simulink model "thrust_torque"  (R2025b)
settings: Solver=VariableStepAuto  StartTime=0.0  StopTime=10.0  RelTol=1e-3
settings Model: Creator=BillL  LastModifiedBy=BillL

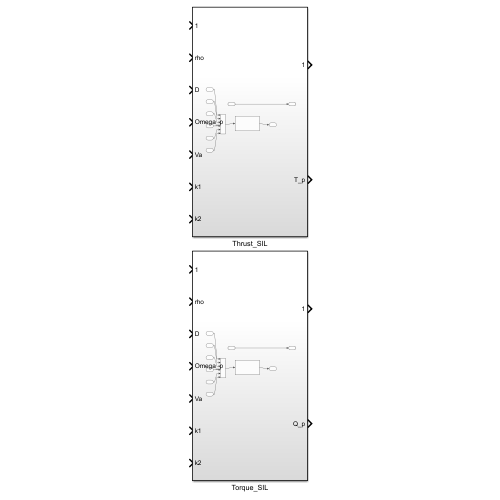
[thumbnail: Simulink's stored preview of the top-level diagram]
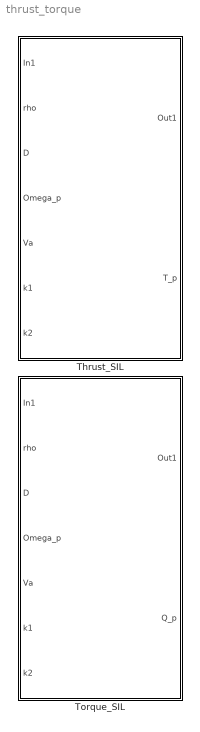
== system thrust_torque ==
  Thrust_SIL : Subsystem
  Torque_SIL : Subsystem

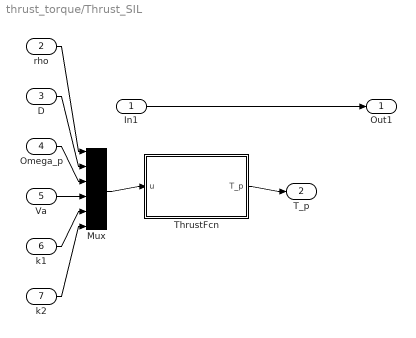
== system thrust_torque/Thrust_SIL ==
  In1 : Inport
  rho : Inport  Port=2
  D : Inport  Port=3
  Omega_p : Inport  Port=4
  Va : Inport  Port=5
  k1 : Inport  Port=6
  k2 : Inport  Port=7
  Mux : Mux  Inputs=6
  ThrustFcn : MATLAB Function  TreatAsAtomicUnit=on
  Out1 : Outport
  T_p : Outport  Port=2
  wires:
  In1/1 -> Out1/1
  rho/1 -> Mux/1
  D/1 -> Mux/2
  Omega_p/1 -> Mux/3
  Va/1 -> Mux/4
  k1/1 -> Mux/5
  k2/1 -> Mux/6
  Mux/1 -> ThrustFcn/1(u)
  ThrustFcn/1(T_p) -> T_p/1

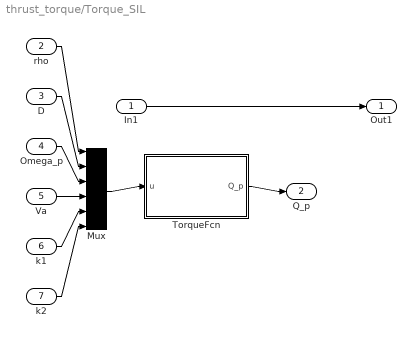
== system thrust_torque/Torque_SIL ==
  In1 : Inport
  rho : Inport  Port=2
  D : Inport  Port=3
  Omega_p : Inport  Port=4
  Va : Inport  Port=5
  k1 : Inport  Port=6
  k2 : Inport  Port=7
  Mux : Mux  Inputs=6
  TorqueFcn : MATLAB Function  TreatAsAtomicUnit=on
  Out1 : Outport
  Q_p : Outport  Port=2
  wires:
  In1/1 -> Out1/1
  rho/1 -> Mux/1
  D/1 -> Mux/2
  Omega_p/1 -> Mux/3
  Va/1 -> Mux/4
  k1/1 -> Mux/5
  k2/1 -> Mux/6
  Mux/1 -> TorqueFcn/1(u)
  TorqueFcn/1(Q_p) -> Q_p/1

== matlab function thrust_torque/Thrust_SIL/ThrustFcn ==
  data: u input; T_p output
function T_p = thrust_block(u)
rho = u(1); D = u(2); Omega_p = u(3); Va = u(4); k1 = u(5); k2 = u(6);
if Omega_p <= 0 || D <= 0
    J = 0; C_T = 0;
else
    J = (2*pi*Va) / (Omega_p*D);
    C_T = k1*J + k2*J^2;
end
T_p = (rho*D^4/(4*pi^2)) * Omega_p^2 * C_T;
end

== matlab function thrust_torque/Torque_SIL/TorqueFcn ==
  data: u input; Q_p output
function Q_p = torque_block(u)
rho = u(1); D = u(2); Omega_p = u(3); Va = u(4); k1 = u(5); k2 = u(6);
if Omega_p <= 0 || D <= 0
    J = 0; C_Q = 0;
else
    J = (2*pi*Va) / (Omega_p*D);
    C_Q = k1*J + k2*J^2;
end
Q_p = (rho*D^5/(4*pi^2)) * Omega_p^2 * C_Q;
end
